simulink model "model"  (R2013a)
settings: Solver=ode45  StartTime=0.0  StopTime=2  RelTol=1e-3
settings Model: Creator=User1  LastModifiedBy=User1

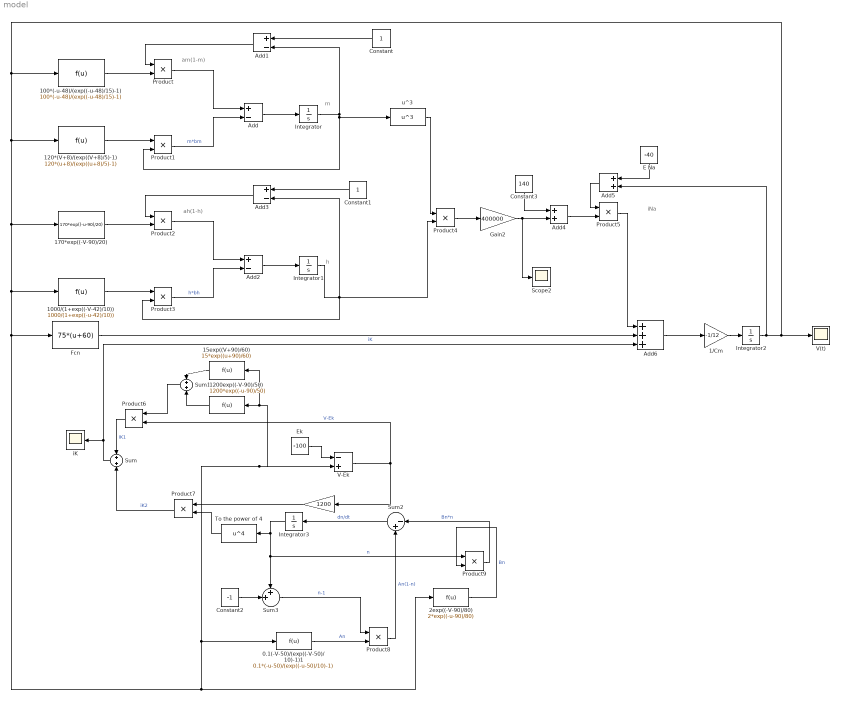
== system model ==
  note: iNa
  note: ah(1-h)
  note: h
  note: am(1-m)
  note: m
  " " : Gain  Gain=1200
  0.1(-V-50)/(exp((-V-50)/10)-1)1 : Fcn  Expr=0.1*(-u-50)/(exp((-u-50)/10)-1)
  1/Cm : Gain  Gain=-1/12
  100*(-u-48)/(exp((-u-48)/15)-1) : Fcn  Expr=100*(-u-48)/(exp((-u-48)/15)-1)
  1000/(1+exp((-V-42)/10)) : Fcn  Expr=1000/(1+exp((-u-42)/10))
  120*(V+8)/(exp((V+8)/5)-1) : Fcn  Expr=120*(u+8)/(exp((u+8)/5)-1)
  1200exp((-V-90)/50) : Fcn  Expr=1200*exp((-u-90)/50)
  15exp((V+90)/60) : Fcn  Expr=15*exp((u+90)/60)
  170*exp((-V-90)/20) : Fcn  Expr=170*exp((-u-90)/20)
  2exp((-V-90)/80) : Fcn  Expr=2*exp((-u-90)/80)
  Add{,1..3} (4 alike) : Sum  Inputs=+-
  Add4 : Sum
  Add5 : Sum
  Add6 : Sum  Inputs=+++
  Constant : Constant
  Constant1 : Constant
  Constant2 : Constant  Value=-1
  Constant3 : Constant  Value=140
  E Na : Constant  Value=-40
  Ek : Constant  Value=-100
  Fcn : Fcn  Expr=75*(u+60)
  Gain2 : Gain  Gain=400000
  Integrator : Integrator  InitialCondition=0.04338  UpperSaturationLimit=500  LowerSaturationLimit=-500
  Integrator1 : Integrator  InitialCondition=0.85218
  Integrator2 : Integrator  InitialCondition=-81.6  UpperSaturationLimit=500  LowerSaturationLimit=-500
  Integrator3 : Integrator  InitialCondition=0.60888  UpperSaturationLimit=1000  LowerSaturationLimit=-1000
  Product{,1..9} (10 alike) : Product
  Scope2 : Scope
      settings: YMin=1.4e+11  YMax=3e+11  SaveName=ScopeData7
  Sum : Sum
  Sum1 : Sum
  Sum2 : Sum  Inputs=|-+
  Sum3 : Sum  Inputs=++|
  To the power of 4 : Fcn  Expr=u^4
  V(t) : Scope
      settings: YMin=39.91  YMax=39.99  SaveName=ScopeData6
  V-Ek : Sum  Inputs=-+
  iK : Scope
      settings: TimeRange=2  YMin=3.325e+15  YMax=3.338e+15  SaveName=ScopeData8
  u^3 : Fcn  Expr=u^3
  wires:
  Integrator2/1 -> 100*(-u-48)/(exp((-u-48)/15)-1)/1, 120*(V+8)/(exp((V+8)/5)-1)/1, 2exp((-V-90)/80)/1, 0.1(-V-50)/(exp((-V-50)/10)-1)1/1, 15exp((V+90)/60)/1, 1200exp((-V-90)/50)/1, V-Ek/2, Fcn/1, 1000/(1+exp((-V-42)/10))/1, 170*exp((-V-90)/20)/1, V(t)/1, Add5/2
  Product3/1 -> Add2/2  "h*bh"
  Product2/1 -> Add2/1
  Add2/1 -> Integrator1/1
  Constant1/1 -> Add3/1
  Add3/1 -> Product2/1
  Integrator1/1 -> Product3/2, Add3/2, Product4/2
  Product1/1 -> Add/2  "m*bm"
  Product/1 -> Add/1
  Add/1 -> Integrator/1
  Constant/1 -> Add1/1
  Add1/1 -> Product/1
  100*(-u-48)/(exp((-u-48)/15)-1)/1 -> Product/2
  120*(V+8)/(exp((V+8)/5)-1)/1 -> Product1/1
  Integrator/1 -> Product1/2, u^3/1, Add1/2
  u^3/1 -> Product4/1
  1000/(1+exp((-V-42)/10))/1 -> Product3/1
  170*exp((-V-90)/20)/1 -> Product2/2
  Product4/1 -> Gain2/1
  Gain2/1 -> Scope2/1, Add4/2
  Constant3/1 -> Add4/1
  Add4/1 -> Product5/2
  Product5/1 -> Add6/1
  1/Cm/1 -> Integrator2/1
  E Na/1 -> Add5/1
  Add5/1 -> Product5/1
  Fcn/1 -> Add6/2
  Add6/1 -> 1/Cm/1
  Product6/1 -> Sum/1  "iK1"
  Product7/1 -> Sum/2  "iK2"
  Ek/1 -> V-Ek/1
  V-Ek/1 -> " "/1, Product6/2  "V-Ek"
  Sum1/1 -> Product6/1
  Sum/1 -> Add6/3, iK/1  "iK"
  1200exp((-V-90)/50)/1 -> Sum1/2
  15exp((V+90)/60)/1 -> Sum1/1
  " "/1 -> Product7/1
  To the power of 4/1 -> Product7/2
  Integrator3/1 -> Sum3/1, Product9/1, To the power of 4/1  "n"
  Sum2/1 -> Integrator3/1  "dn/dt"
  Constant2/1 -> Sum3/2
  Sum3/1 -> Product8/1  "n-1"
  0.1(-V-50)/(exp((-V-50)/10)-1)1/1 -> Product8/2  "An"
  Product8/1 -> Sum2/2  "An(1-n)"
  2exp((-V-90)/80)/1 -> Product9/2  "Bn"
  Product9/1 -> Sum2/1  "Bn*n"
